simulink model "pendulo_simples"  (R2018b)
settings: Solver=VariableStepAuto  StartTime=0.0  StopTime=10.0  RelTol=1e-3
values from neighbouring files (symbols this model uses):
  A = double(subs(A,[h,u],[heq,ueq]))    [tanque_simples.m]
  B = double(subs(B,[h,u],[heq,ueq]))    [tanque_simples.m]
  ueq = double(solve(subs(f==0,h,heq),u))    [tanque_simples.m]
undefined symbols (not defined in the file or in its folder): uop, xeq
settings Model: Creator=bernardo  LastModifiedBy=bernardo

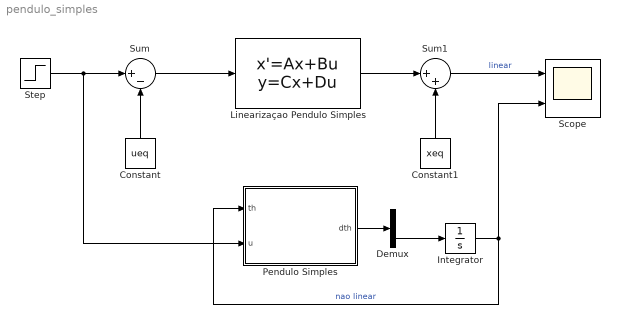
== system pendulo_simples ==
  Constant : Constant  Value=ueq
  Constant1 : Constant  Value=xeq
  Demux : Demux  Outputs=2
  Integrator : Integrator
  Linearizaçao Pendulo Simples : StateSpace  A=A  B=B  C=[1, 0]  D=0  InitialCondition=0
  Pendulo Simples : MATLAB Function  TreatAsAtomicUnit=on
  Scope : Scope  NumInputPorts=2
  Step : Step  Time=0  After=1*uop  SampleTime=0
  Sum : Sum  Inputs=|+-
  Sum1 : Sum  Inputs=|++
  wires:
  Integrator/1 -> Scope/2, Pendulo Simples/1(th)  "nao linear"
  Sum/1 -> Linearizaçao Pendulo Simples/1
  Sum1/1 -> Scope/1  "linear"
  Constant1/1 -> Sum1/2
  Constant/1 -> Sum/2
  Step/1 -> Pendulo Simples/2(u), Sum/1
  Linearizaçao Pendulo Simples/1 -> Sum1/1
  Pendulo Simples/1(dth) -> Demux/1
  Demux/2 -> Integrator/1

== matlab function pendulo_simples/Pendulo Simples ==
  data: th input; u input; dth output
function dth = fcn(th,u)
m = 1;
k = 1;
g = 9.8;
dth = zeros(2,1);
dth(1) = dth(2);
dth(2) = u/m - k/m - g*sin(dth(1));
end
